simulink subsystem "DcDcConverterBasic_refsub"  (R2020b)
settings: Solver=VariableStepAuto  StartTime=0.0  StopTime=10.0  RelTol=1e-3
undefined symbols (not defined in the file): Minus, Plus
libraries: fl_lib x8, nesl_utility x6
settings Model: Creator=isaacito  LastModifiedBy=isaacito

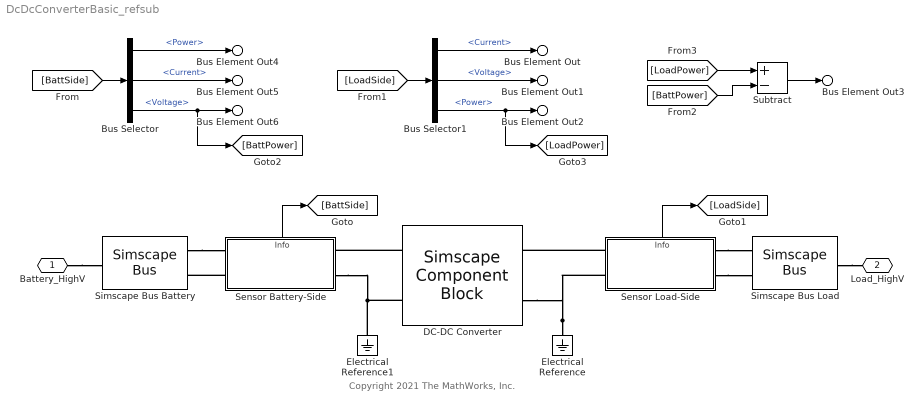
== system DcDcConverterBasic_refsub ==
  note: Copyright 2021 The MathWorks, Inc.
  Bus Selector : BusSelector  OutputSignals=Power,Current,Voltage
  Bus Selector1 : BusSelector  OutputSignals=Current,Voltage,Power
  DC-DC Converter : SimscapeComponentBlock  SourceFile=DcDcConverterCustom  ComponentPath=DcDcConverterCustom  ComponentVariants="[\"DcDcConverterCustom\"]"  ComponentVariantNames="[\"DcDcConverterCustom\"]"  ClassName=DcDcConverterCustom  SchemaVersion=1  v_ref=dcDcConverter.outputVoltageRef_V V  P_rated=dcDcConverter.outputPower_kW kW  eff_pct=dcDcConverter.efficiency_pct  P_fixed=dcDcConverter.fixedLoss_W W  tau=dcDcConverter.timeConstant_s s  i_batt_max=500 A
      settings: CopyFcn=simscape.engine.sli.internal.componentblockcallback(gcbh,'COPY')  PreCopyFcn=simscape.engine.sli.internal.componentblockcallback(gcbh,'PRECOPY')  PreDeleteFcn=simscape.engine.sli.internal.componentblockcallback(gcbh,'PREDELETE')  LogSimulationData=on  InternalSimscapePortConfiguration="{\"Bottom\":[],\"Left\":[{\"id\":\"p_batt\",\"label\":\"B+\",\"type\":\"foundation.electrical.electrical\"},{\"id\":\"n_batt\",\"label\":\"B-\",\"type\":\"foundation.electrical.electrical\"}],\"Right\":[{\"id\":\"p_load\",\"label\":\"L+\",\"type\":\"foundation.electrical.electrical\"},{\"id\":\"n_load\",\"label\":\"L-\",\"type\":\"foundation.electrical.electrical\"}],\"Top\":[]}"
      mask Type: Simple DC-DC Converter
  Electrical Reference : fl_lib/Electrical/Electrical Elements/Electrical Reference
  Electrical Reference1 : fl_lib/Electrical/Electrical Elements/Electrical Reference
  Sensor Battery-Side : Subsystem
      settings: PortSchema="{\"entries\":[{\"content\":{\"sides\":[{\"content\":{\"connectorIds\":[\"LConn1\",\"LConn2\"]},\"type\":\"ConnectorPlacement.EquallySpacedRectSide\",\"uuid\":\"30a3c46a-b3e0-427d-a0c9-e296da4172be\"},{\"content\":{\"connectorIds\":[\"RConn1\",\"RConn2\"],\"side\":\"RIGHT\"},\"type\":\"ConnectorPlacement.EquallySpacedRectSide\",\"uuid\":\"48782190-a487-49f7-9f54-e3a703410830\"},{\"content\":{\"connectorIds\":[\"Out1\"],\"side\":\"TOP\"},\"type\":\"ConnectorPlacement.EquallySpacedRectSide\",\"uuid\":\"37a901e6-af8d-4d93-a097-cadde85f702b\"},{\"content\":{\"connectorIds\":[],\"side\":\"HIDDEN\"},\"type\":\"ConnectorPlacement.EquallySpacedRectSide\",\"uuid\":\"e05a31e4-ac96-47b1-b0f8-1d500f120ecd\"}]},\"type\":\"ConnectorPlacement.EquallySpacedConnector\",\"uuid\":\"392c062c-c64b-4158-94e7-7a4212c653a5\"}],\"packageUris\":[\"http://schema.mathworks.com/mf0/Connector/R2020b\"],\"version\":\"1.0\"}"
  Sensor Load-Side : Subsystem
      settings: PortSchema="{\"entries\":[{\"content\":{\"sides\":[{\"content\":{\"connectorIds\":[\"LConn1\",\"LConn2\"]},\"type\":\"ConnectorPlacement.EquallySpacedRectSide\",\"uuid\":\"30a3c46a-b3e0-427d-a0c9-e296da4172be\"},{\"content\":{\"connectorIds\":[\"RConn1\",\"RConn2\"],\"side\":\"RIGHT\"},\"type\":\"ConnectorPlacement.EquallySpacedRectSide\",\"uuid\":\"48782190-a487-49f7-9f54-e3a703410830\"},{\"content\":{\"connectorIds\":[\"Out1\"],\"side\":\"TOP\"},\"type\":\"ConnectorPlacement.EquallySpacedRectSide\",\"uuid\":\"37a901e6-af8d-4d93-a097-cadde85f702b\"},{\"content\":{\"connectorIds\":[],\"side\":\"HIDDEN\"},\"type\":\"ConnectorPlacement.EquallySpacedRectSide\",\"uuid\":\"e05a31e4-ac96-47b1-b0f8-1d500f120ecd\"}]},\"type\":\"ConnectorPlacement.EquallySpacedConnector\",\"uuid\":\"392c062c-c64b-4158-94e7-7a4212c653a5\"}],\"packageUris\":[\"http://schema.mathworks.com/mf0/Connector/R2020b\"],\"version\":\"1.0\"}"
  Simscape Bus Battery : SimscapeBus  HierarchyStrings=Plus;Minus
  Simscape Bus Load : SimscapeBus  HierarchyStrings=Plus;Minus
  Subtract : Sum  Inputs=+-
  Battery_HighV : PMIOPort  Side=Left
  Load_HighV : PMIOPort  Port=2  Side=Right
  Bus Element Out : Outport  PortName=Info  Element=LoadCurr
  Bus Element Out1 : Outport  PortName=Info  Element=LoadV
  Bus Element Out2 : Outport  PortName=Info  Element=LoadPower
  Bus Element Out3 : Outport  PortName=Info  Element=PowerDiff
  Bus Element Out4 : Outport  PortName=Info  Element=BattPower
  Bus Element Out5 : Outport  PortName=Info  Element=BattCurr
  Bus Element Out6 : Outport  PortName=Info  Element=BattV
  wires:
  Sensor Battery-Side/1(Info) -> [BattSide]
  Sensor Load-Side/1(Info) -> [LoadSide]
  [BattSide] -> Bus Selector/1
  [LoadSide] -> Bus Selector1/1
  Bus Selector1/1 -> Bus Element Out/1  "<Current>"
  Bus Selector1/2 -> Bus Element Out1/1  "<Voltage>"
  Bus Selector1/3 -> Bus Element Out2/1, [LoadPower]  "<Power>"
  Bus Selector/1 -> Bus Element Out4/1  "<Power>"
  Bus Selector/2 -> Bus Element Out5/1  "<Current>"
  Bus Selector/3 -> Bus Element Out6/1, [BattPower]  "<Voltage>"
  Subtract/1 -> Bus Element Out3/1
  [BattPower] -> Subtract/2
  [LoadPower] -> Subtract/1
  connections:
  DC-DC Converter/LConn2 -- Electrical Reference1/LConn1 -- Sensor Battery-Side/RConn2
  Electrical Reference/LConn1 -- Sensor Load-Side/LConn2 -- DC-DC Converter/RConn2
  Battery_HighV/RConn1 -- Simscape Bus Battery/RConn1
  Simscape Bus Load/RConn1 -- Load_HighV/RConn1
  DC-DC Converter/LConn1 -- Sensor Battery-Side/RConn1
  Simscape Bus Battery/LConn1 -- Sensor Battery-Side/LConn1
  Sensor Battery-Side/LConn2 -- Simscape Bus Battery/LConn2
  Sensor Load-Side/LConn1 -- DC-DC Converter/RConn1
  Sensor Load-Side/RConn1 -- Simscape Bus Load/LConn1
  Sensor Load-Side/RConn2 -- Simscape Bus Load/LConn2

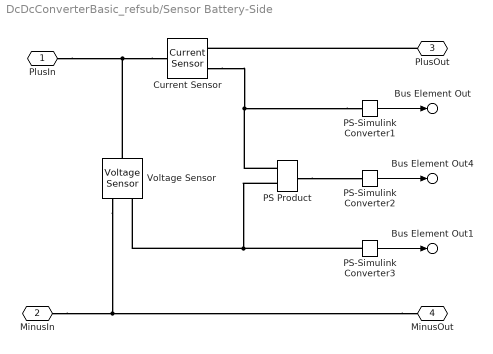
== system DcDcConverterBasic_refsub/Sensor Battery-Side ==
  Current Sensor : fl_lib/Electrical/Electrical Sensors/Current Sensor
  PS Product : fl_lib/Physical Signals/Functions/PS Product
  PS-Simulink Converter1 : nesl_utility/PS-Simulink Converter  PhysicalDomain=network_engine_domain  SubClassName=ps_output  LeftPortType=input  RightPortType=output  PseudoPeriodic=off  Frequencies=[]  Unit=A  AffineConversion=off
  PS-Simulink Converter2 : nesl_utility/PS-Simulink Converter  PhysicalDomain=network_engine_domain  SubClassName=ps_output  LeftPortType=input  RightPortType=output  PseudoPeriodic=off  Frequencies=[]  Unit=kW  AffineConversion=off
  PS-Simulink Converter3 : nesl_utility/PS-Simulink Converter  PhysicalDomain=network_engine_domain  SubClassName=ps_output  LeftPortType=input  RightPortType=output  PseudoPeriodic=off  Frequencies=[]  Unit=V  AffineConversion=off
  Voltage Sensor : fl_lib/Electrical/Electrical Sensors/Voltage Sensor
  PlusIn : PMIOPort  Side=Left
  MinusIn : PMIOPort  Port=2  Side=Left
  PlusOut : PMIOPort  Port=3  Side=Right
  MinusOut : PMIOPort  Port=4  Side=Right
  Bus Element Out : Outport  PortName=Info  Element=Current
  Bus Element Out1 : Outport  PortName=Info  Element=Voltage
  Bus Element Out4 : Outport  PortName=Info  Element=Power
  wires:
  PS-Simulink Converter1/1 -> Bus Element Out/1
  PS-Simulink Converter3/1 -> Bus Element Out1/1
  PS-Simulink Converter2/1 -> Bus Element Out4/1
  connections:
  PS-Simulink Converter1/LConn1 -- PS Product/LConn1 -- Current Sensor/RConn1
  MinusOut/RConn1 -- Voltage Sensor/RConn2 -- MinusIn/RConn1
  Current Sensor/LConn1 -- Voltage Sensor/LConn1 -- PlusIn/RConn1
  PlusOut/RConn1 -- Current Sensor/RConn2
  Voltage Sensor/RConn1 -- PS Product/LConn2 -- PS-Simulink Converter3/LConn1
  PS Product/RConn1 -- PS-Simulink Converter2/LConn1

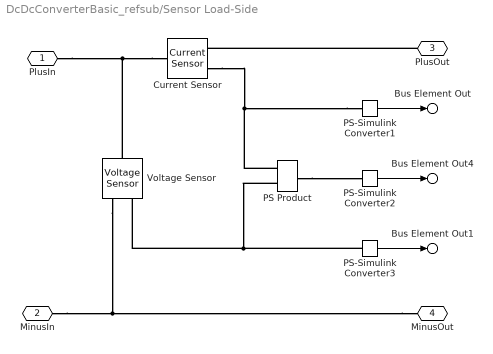
== system DcDcConverterBasic_refsub/Sensor Load-Side ==
  Current Sensor : fl_lib/Electrical/Electrical Sensors/Current Sensor
  PS Product : fl_lib/Physical Signals/Functions/PS Product
  PS-Simulink Converter1 : nesl_utility/PS-Simulink Converter  PhysicalDomain=network_engine_domain  SubClassName=ps_output  LeftPortType=input  RightPortType=output  PseudoPeriodic=off  Frequencies=[]  Unit=A  AffineConversion=off
  PS-Simulink Converter2 : nesl_utility/PS-Simulink Converter  PhysicalDomain=network_engine_domain  SubClassName=ps_output  LeftPortType=input  RightPortType=output  PseudoPeriodic=off  Frequencies=[]  Unit=kW  AffineConversion=off
  PS-Simulink Converter3 : nesl_utility/PS-Simulink Converter  PhysicalDomain=network_engine_domain  SubClassName=ps_output  LeftPortType=input  RightPortType=output  PseudoPeriodic=off  Frequencies=[]  Unit=V  AffineConversion=off
  Voltage Sensor : fl_lib/Electrical/Electrical Sensors/Voltage Sensor
  PlusIn : PMIOPort  Side=Left
  MinusIn : PMIOPort  Port=2  Side=Left
  PlusOut : PMIOPort  Port=3  Side=Right
  MinusOut : PMIOPort  Port=4  Side=Right
  Bus Element Out : Outport  PortName=Info  Element=Current
  Bus Element Out1 : Outport  PortName=Info  Element=Voltage
  Bus Element Out4 : Outport  PortName=Info  Element=Power
  wires:
  PS-Simulink Converter1/1 -> Bus Element Out/1
  PS-Simulink Converter3/1 -> Bus Element Out1/1
  PS-Simulink Converter2/1 -> Bus Element Out4/1
  connections:
  PS-Simulink Converter1/LConn1 -- PS Product/LConn1 -- Current Sensor/RConn1
  MinusOut/RConn1 -- Voltage Sensor/RConn2 -- MinusIn/RConn1
  Current Sensor/LConn1 -- Voltage Sensor/LConn1 -- PlusIn/RConn1
  PlusOut/RConn1 -- Current Sensor/RConn2
  Voltage Sensor/RConn1 -- PS Product/LConn2 -- PS-Simulink Converter3/LConn1
  PS Product/RConn1 -- PS-Simulink Converter2/LConn1
